simulink model "sldemo_drivingcycle"  (R2019b)
settings: Solver=ode45  StartTime=0.0  StopTime=1e5  MaxStep=1  RelTol=1e-3  EnableMultiTasking=on
libraries: drivingcycle_lib x1
settings Model: Creator=e102261  LastModifiedBy=hoyeonjigi
settings DataIOCC: LimitDataPoints=on  SaveFormat=Array  SaveOutput=off  SignalLogging=off  DSMLogging=off  SaveTime=off  ReturnWorkspaceOutputs=off
settings OptimizationCC: ExpressionDepthLimit=2147483647  LifeSpan=inf
settings DebuggingCC: UnderspecifiedInitializationDetection=Classic  MergeDetectMultiDrivingBlocksExec=none  SolverPrmCheckMsg=warning  MultiTaskDSMMsg=warning  MultiTaskCondExecSysMsg=none  FcnCallInpInsideContextMsg=warning  StateNameClashWarn=warning  SFUnexpectedBacktrackingDiag=warning  SFNoUnconditionalDefaultTransitionDiag=warning  SFExecutionAtInitializationDiag=none  ArithmeticOperatorsInVariantConditions=warning
settings HardwareCC: ProdBitPerPointer=32  ProdBitPerSizeT=32  ProdBitPerPtrDiffT=32  ProdLargestAtomicFloat=None  ProdIntDivRoundTo=Undefined  ProdEndianess=Unspecified  ProdWordSize=32  ProdHWDeviceType=32-bit Generic
settings ModelReferenceCC: PropagateSignalLabelsOutOfModel=off
settings SFSimCC: SimUseLocalCustomCode=off  CustomCodeUndefinedFunction=UseInterfaceOnly
settings RTWCC: RTWUseLocalCustomCode=off
settings CodeAppCC: StateflowObjectComments=on
settings GRTTargetCC: TargetLangStandard=C89/C90 (ANSI)
settings ConfigComp: CovMetricSettings=dw  CovHtmlReporting=on  CovSaveCumulativeToWorkspaceVar=on  CovSaveSingleToWorkspaceVar=on  CovExternalEMLEnable=off

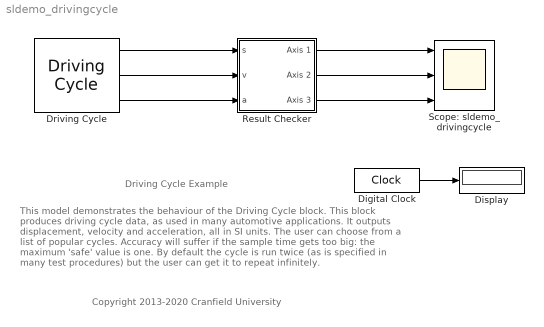
== system sldemo_drivingcycle ==
  note: This model demonstrates the behaviour of the Driving Cycle block.  This block
      | produces driving cycle data, as used in many automotive applications.  It
      | outputs displacement, velocity and acceleration, all in SI units.  The user can
      | choose from a list of popular cycles. Accuracy will suffer if the sample time gets
      | too big: the maximum 'safe' value is one.  By default the cycle is run twice (as
      | is specified in many test procedures) but the user can get it to repeat infinitely.
  note: Driving Cycle Example
  note: Copyright 2013-2020 Cranfield University
  Digital Clock : DigitalClock
  Display : Display
  Driving Cycle : drivingcycle_lib/Driving Cycle  CycleName=WLTP class 3  CycleRepeatsForever=off
      settings: SourceProductName=Driving Cycle Blockset
  Result Checker : Subsystem
  Scope: sldemo_drivingcycle : Scope  NumInputPorts=3
      settings: AttributesFormatString=|
      | please use scope's axis autoscaling
      | button after simulation
  wires:
  Result Checker/1(Axis 1) -> Scope: sldemo_drivingcycle/1
  Result Checker/2(Axis 2) -> Scope: sldemo_drivingcycle/2
  Result Checker/3(Axis 3) -> Scope: sldemo_drivingcycle/3
  Digital Clock/1 -> Display/1
  Driving Cycle/1 -> Result Checker/1(s)
  Driving Cycle/2 -> Result Checker/2(v)
  Driving Cycle/3 -> Result Checker/3(a)

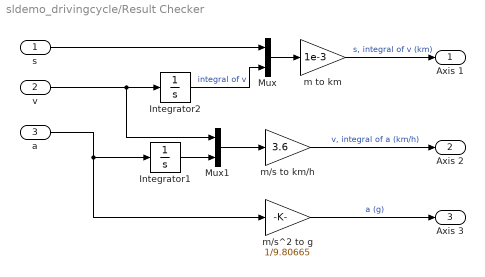
== system sldemo_drivingcycle/Result Checker ==
  s : Inport
  v : Inport  Port=2
  a : Inport  Port=3
  Integrator1 : Integrator
  Integrator2 : Integrator
  Mux : Mux  Inputs=2
  Mux1 : Mux  Inputs=2
  m to km : Gain  Gain=1e-3
  m/s to km/h : Gain  Gain=3.6
  m/s^2 to g : Gain  Gain=1/9.80665
  Axis 1 : Outport
  Axis 2 : Outport  Port=2
  Axis 3 : Outport  Port=3
  wires:
  Mux/1 -> m to km/1
  Integrator1/1 -> Mux1/2
  Integrator2/1 -> Mux/2  "integral of v"
  Mux1/1 -> m/s to km/h/1
  v/1 -> Integrator2/1, Mux1/1
  a/1 -> m/s^2 to g/1, Integrator1/1
  s/1 -> Mux/1
  m to km/1 -> Axis 1/1  "s, integral of v (km)"
  m/s to km/h/1 -> Axis 2/1  "v, integral of a (km/h)"
  m/s^2 to g/1 -> Axis 3/1  "a (g)"
